simulink model "BUILDmod1"  (Simulink 5.0)
settings: Solver=ode23tb  StartTime=0  StopTime=20*24*3600  MaxStep=900  RelTol=1e-3
settings Model: LastModifiedBy=bwjosvs  ExtModeTrigMode=oneshot  ExtModeArmWhenConnect=off  LimitDataPoints=off  BooleanDataType=off

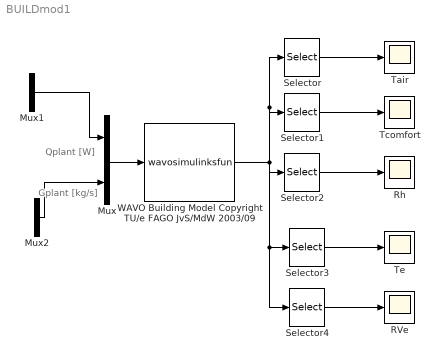
== system BUILDmod1 ==
  note: Qplant [W]
  note: Gplant [kg/s]
  Mux : Mux  Inputs=2
  Mux1 : Mux
  Mux2 : Mux
  RVe : Scope
      settings: YMin=0  YMax=11  SaveName=Rhe
  Rh : Scope
      settings: TimeRange=1728000  YMin=0.5750000000000001  YMax=0.7750000000000001  SaveName=Rh
  Selector : Selector  Elements=[1:4]  InputPortWidth=14
  Selector1 : Selector  Elements=4+[1:4]  InputPortWidth=14
  Selector2 : Selector  Elements=8+[1:4]  InputPortWidth=14
  Selector3 : Selector  Elements=13  InputPortWidth=14
  Selector4 : Selector  Elements=14  InputPortWidth=14
  Tair : Scope
      settings: YMin=6.5  YMax=14  SaveName=Tair
  Tcomfort : Scope
      settings: YMin=8.5  YMax=14.5  SaveName=Tcom
  Te : Scope
      settings: YMin=0  YMax=11  SaveName=Te
  WAVO Building Model Copyright TU/e FAGO JvS/MdW 2003/09 : S-Function  FunctionName=wavosimulinksfun  Parameters=Filename  mask{Filename='Buildingm1'}
      mask prompts: Filename "Enter Inputfile between ' ' and without .m :"
      mask Display: image(imread('fagologo.jpg'))
  wires:
  Mux/1 -> WAVO Building Model Copyright TU/e FAGO JvS/MdW 2003/09/1
  WAVO Building Model Copyright TU/e FAGO JvS/MdW 2003/09/1 -> Selector/1, Selector1/1, Selector2/1, Selector3/1, Selector4/1
  Selector/1 -> Tair/1
  Selector1/1 -> Tcomfort/1
  Selector2/1 -> Rh/1
  Selector3/1 -> Te/1
  Selector4/1 -> RVe/1
  Mux1/1 -> Mux/1
  Mux2/1 -> Mux/2
